simulink model "AFS_VDDrftComp"  (R2016b)
settings: configuration reference "CodeGenConfigSet" (kept outside this file)
values from neighbouring files (symbols this model uses):
  AFS_aOvrnAdjMax_C = Calibration.Parameter    [init_AFS_VDDrftComp.m]    (also in init_AFS_VDDrftComp_SIL.m = Simulink.Parameter)
  AFS_aOvrnAdjMin_C = Calibration.Parameter    [init_AFS_VDDrftComp.m]    (also in init_AFS_VDDrftComp_SIL.m = Simulink.Parameter)
  AFS_dmIdlAirMsLim_C = Calibration.Parameter    [init_AFS_VDDrftComp.m]    (also in init_AFS_VDDrftComp_SIL.m = Simulink.Parameter)
  AFS_dmLdAirMsLim_C = Calibration.Parameter    [init_AFS_VDDrftComp.m]    (also in init_AFS_VDDrftComp_SIL.m = Simulink.Parameter)
  AFS_dnEngLdAdjThresHi_C = Calibration.Parameter    [init_AFS_VDDrftComp.m]    (also in init_AFS_VDDrftComp_SIL.m = Simulink.Parameter)
  AFS_dpLdAdjThresHi_C = Calibration.Parameter    [init_AFS_VDDrftComp.m]    (also in init_AFS_VDDrftComp_SIL.m = Simulink.Parameter)
  AFS_dqLdAdjThresHi_C = Calibration.Parameter    [init_AFS_VDDrftComp.m]    (also in init_AFS_VDDrftComp_SIL.m = Simulink.Parameter)
  AFS_drWtPenDetThresHi_C = Calibration.Parameter    [init_AFS_VDDrftComp.m]    (also in init_AFS_VDDrftComp_SIL.m = Simulink.Parameter)
  AFS_facAdjPlausDiff_C = Calibration.Parameter    [init_AFS_VDDrftComp.m]    (also in init_AFS_VDDrftComp_SIL.m = Simulink.Parameter)
  AFS_facAirMsPT1_C = Calibration.Parameter    [init_AFS_VDDrftComp.m]    (also in init_AFS_VDDrftComp_SIL.m = Simulink.Parameter)
  AFS_facBstPresPT1_C = Calibration.Parameter    [init_AFS_VDDrftComp.m]    (also in init_AFS_VDDrftComp_SIL.m = Simulink.Parameter)
  AFS_facCorExtpIdl_CUR = Calibration.Parameter    [init_AFS_VDDrftComp.m]    (also in init_AFS_VDDrftComp_SIL.m = Simulink.Parameter)
  AFS_facCorExtpIdl_CURX = Calibration.Parameter    [init_AFS_VDDrftComp.m]    (also in init_AFS_VDDrftComp_SIL.m = Simulink.Parameter)
  AFS_facCorExtpLd_CUR = Calibration.Parameter    [init_AFS_VDDrftComp.m]    (also in init_AFS_VDDrftComp_SIL.m = Simulink.Parameter)
  AFS_facCorExtpLd_CURX = Calibration.Parameter    [init_AFS_VDDrftComp.m]    (also in init_AFS_VDDrftComp_SIL.m = Simulink.Parameter)
  AFS_facCorFacPT1_C = Calibration.Parameter    [init_AFS_VDDrftComp.m]    (also in init_AFS_VDDrftComp_SIL.m = Simulink.Parameter)
  AFS_facIdlAdjPlausMax_C = Calibration.Parameter    [init_AFS_VDDrftComp.m]    (also in init_AFS_VDDrftComp_SIL.m = Simulink.Parameter)
  AFS_facIdlAdjValMax_C = Calibration.Parameter    [init_AFS_VDDrftComp.m]    (also in init_AFS_VDDrftComp_SIL.m = Simulink.Parameter)
  AFS_facIdlAdjValMin_C = Calibration.Parameter    [init_AFS_VDDrftComp.m]    (also in init_AFS_VDDrftComp_SIL.m = Simulink.Parameter)
  AFS_facIdlAdjValStepLim_C = Calibration.Parameter    [init_AFS_VDDrftComp.m]    (also in init_AFS_VDDrftComp_SIL.m = Simulink.Parameter)
  AFS_facLdAdjPlausMin_C = Calibration.Parameter    [init_AFS_VDDrftComp.m]    (also in init_AFS_VDDrftComp_SIL.m = Simulink.Parameter)
  AFS_facLdAdjValMax_C = Calibration.Parameter    [init_AFS_VDDrftComp.m]    (also in init_AFS_VDDrftComp_SIL.m = Simulink.Parameter)
  AFS_facLdAdjValMin_C = Calibration.Parameter    [init_AFS_VDDrftComp.m]    (also in init_AFS_VDDrftComp_SIL.m = Simulink.Parameter)
  AFS_facLdAdjValStepLim_C = Calibration.Parameter    [init_AFS_VDDrftComp.m]    (also in init_AFS_VDDrftComp_SIL.m = Simulink.Parameter)
  AFS_facLoThresIdlAdjVal_C = Calibration.Parameter    [init_AFS_VDDrftComp.m]    (also in init_AFS_VDDrftComp_SIL.m = Simulink.Parameter)
  AFS_facLoThresLdAdjVal_C = Calibration.Parameter    [init_AFS_VDDrftComp.m]    (also in init_AFS_VDDrftComp_SIL.m = Simulink.Parameter)
  AFS_facnEngPT1_C = Calibration.Parameter    [init_AFS_VDDrftComp.m]    (also in init_AFS_VDDrftComp_SIL.m = Simulink.Parameter)
  AFS_facQntCurrPT1_C = Calibration.Parameter    [init_AFS_VDDrftComp.m]    (also in init_AFS_VDDrftComp_SIL.m = Simulink.Parameter)
  AFS_facWtPenDetPT1_C = Calibration.Parameter    [init_AFS_VDDrftComp.m]    (also in init_AFS_VDDrftComp_SIL.m = Simulink.Parameter)
  AFS_nAvrgIdlAdjThresHi_C = Calibration.Parameter    [init_AFS_VDDrftComp.m]    (also in init_AFS_VDDrftComp_SIL.m = Simulink.Parameter)
  AFS_nAvrgIdlAdjThresLo_C = Calibration.Parameter    [init_AFS_VDDrftComp.m]    (also in init_AFS_VDDrftComp_SIL.m = Simulink.Parameter)
  AFS_nOvrnAdjMax_C = Calibration.Parameter    [init_AFS_VDDrftComp.m]    (also in init_AFS_VDDrftComp_SIL.m = Simulink.Parameter)
  AFS_nOvrnAdjMin_C = Calibration.Parameter    [init_AFS_VDDrftComp.m]    (also in init_AFS_VDDrftComp_SIL.m = Simulink.Parameter)
  AFS_numAirDrftComp_C = Calibration.Parameter    [init_AFS_VDDrftComp.m]    (also in init_AFS_VDDrftComp_SIL.m = Simulink.Parameter)
  AFS_numEnvTemp_C = Calibration.Parameter    [init_AFS_VDDrftComp.m]    (also in init_AFS_VDDrftComp_SIL.m = Simulink.Parameter)
  AFS_numOvrnAdjGearMin_C = Calibration.Parameter    [init_AFS_VDDrftComp.m]    (also in init_AFS_VDDrftComp_SIL.m = Simulink.Parameter)
  AFS_pBstAtmDiffLim_C = Calibration.Parameter    [init_AFS_VDDrftComp.m]    (also in init_AFS_VDDrftComp_SIL.m = Simulink.Parameter)
  AFS_pBstLdAdjThresHi_C = Calibration.Parameter    [init_AFS_VDDrftComp.m]    (also in init_AFS_VDDrftComp_SIL.m = Simulink.Parameter)
  AFS_pBstLdAdjThresLo_C = Calibration.Parameter    [init_AFS_VDDrftComp.m]    (also in init_AFS_VDDrftComp_SIL.m = Simulink.Parameter)
  AFS_qCurrIdlAdjThresHi_C = Calibration.Parameter    [init_AFS_VDDrftComp.m]    (also in init_AFS_VDDrftComp_SIL.m = Simulink.Parameter)
  AFS_qCurrIdlAdjThresLo_C = Calibration.Parameter    [init_AFS_VDDrftComp.m]    (also in init_AFS_VDDrftComp_SIL.m = Simulink.Parameter)
  AFS_qWinLdAdjThresHi_CUR = Calibration.Parameter    [init_AFS_VDDrftComp.m]    (also in init_AFS_VDDrftComp_SIL.m = Simulink.Parameter)
  AFS_qWinLdAdjThresHi_CURX = Calibration.Parameter    [init_AFS_VDDrftComp.m]    (also in init_AFS_VDDrftComp_SIL.m = Simulink.Parameter)
  AFS_qWinLdAdjThresLo_CUR = Calibration.Parameter    [init_AFS_VDDrftComp.m]    (also in init_AFS_VDDrftComp_SIL.m = Simulink.Parameter)
  AFS_qWinLdAdjThresLo_CURX = Calibration.Parameter    [init_AFS_VDDrftComp.m]    (also in init_AFS_VDDrftComp_SIL.m = Simulink.Parameter)
  AFS_swtAdjPlausLim_C = Calibration.Parameter    [init_AFS_VDDrftComp.m]    (also in init_AFS_VDDrftComp_SIL.m = Simulink.Parameter)
  AFS_swtAirMsCorRls_C = Calibration.Parameter    [init_AFS_VDDrftComp.m]    (also in init_AFS_VDDrftComp_SIL.m = Simulink.Parameter)
  AFS_swtLdAdjSel_C = Calibration.Parameter    [init_AFS_VDDrftComp.m]    (also in init_AFS_VDDrftComp_SIL.m = Simulink.Parameter)
  AFS_tAirAdjRlsThresHi_C = Calibration.Parameter    [init_AFS_VDDrftComp.m]    (also in init_AFS_VDDrftComp_SIL.m = Simulink.Parameter)
  AFS_tAirAdjRlsThresLo_C = Calibration.Parameter    [init_AFS_VDDrftComp.m]    (also in init_AFS_VDDrftComp_SIL.m = Simulink.Parameter)
  AFS_tEnvAdjRlsThresHi_C = Calibration.Parameter    [init_AFS_VDDrftComp.m]    (also in init_AFS_VDDrftComp_SIL.m = Simulink.Parameter)
  AFS_tEnvAdjRlsThresLo_C = Calibration.Parameter    [init_AFS_VDDrftComp.m]    (also in init_AFS_VDDrftComp_SIL.m = Simulink.Parameter)
  AFS_tiAdjRlsDel_C = Calibration.Parameter    [init_AFS_VDDrftComp.m]    (also in init_AFS_VDDrftComp_SIL.m = Simulink.Parameter)
  AFS_tiIdlAdjRlsDeb = Calibration.Parameter    [init_AFS_VDDrftComp.m]    (also in init_AFS_VDDrftComp_SIL.m = Simulink.Parameter)
  AFS_tiLdAdjRlsDeb = Calibration.Parameter    [init_AFS_VDDrftComp.m]    (also in init_AFS_VDDrftComp_SIL.m = Simulink.Parameter)
  AFS_tiStrtDelAdjRls_C = Calibration.Parameter    [init_AFS_VDDrftComp.m]    (also in init_AFS_VDDrftComp_SIL.m = Simulink.Parameter)
  AFS_tiWtPenDeb = Calibration.Parameter    [init_AFS_VDDrftComp.m]    (also in init_AFS_VDDrftComp_SIL.m = Simulink.Parameter)
  AFS_vOvrnAdjMin_C = Calibration.Parameter    [init_AFS_VDDrftComp.m]    (also in init_AFS_VDDrftComp_SIL.m = Simulink.Parameter)
  AFS_vVehLdAdjThresHi_C = Calibration.Parameter    [init_AFS_VDDrftComp.m]    (also in init_AFS_VDDrftComp_SIL.m = Simulink.Parameter)
  AFS_vVehLdAdjThresLo_C = Calibration.Parameter    [init_AFS_VDDrftComp.m]    (also in init_AFS_VDDrftComp_SIL.m = Simulink.Parameter)
  AIRCTL_DRFTCOMP = fi(5,State_uint8)    [init_AFS_VDDrftComp.m]    (also in init_AFS_VDDrftComp_SIL.m)
undefined symbols (not defined in the file or in its folder): AFS_VDDrftComp_DT, Switch_conv
libraries: simulink x82, CXLib x13
(part 1 of 2)
settings Model: Creator=Colin  LastModifiedBy=guanxiaoxing
settings ConfigSetRef: SourceLocation=Base Workspace

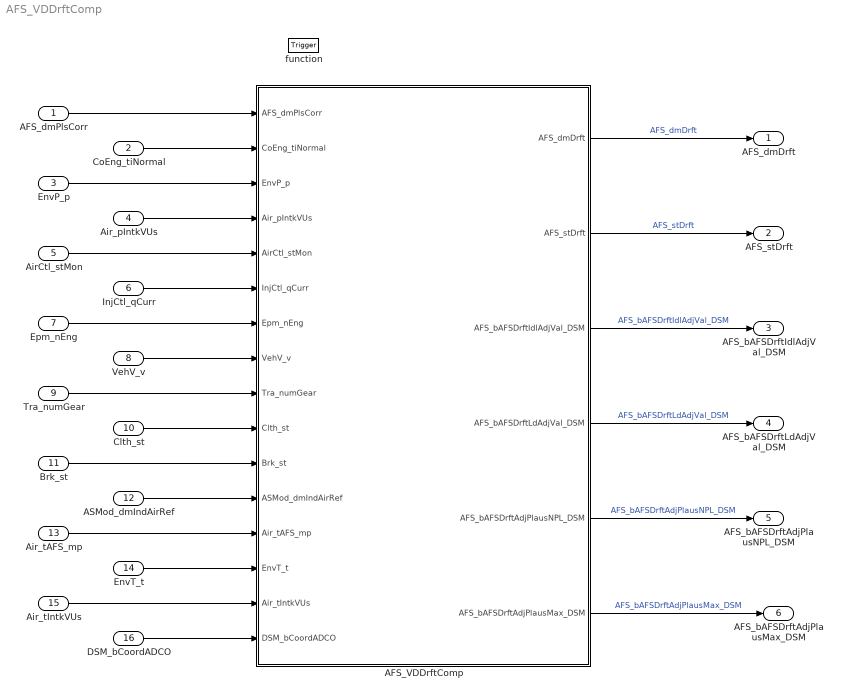
== system AFS_VDDrftComp ==
  AFS_dmPlsCorr : Inport  Tag=kg/h  Description=Pulsation corrected air mass.  OutMin=-8192  OutMax=8191  OutDataTypeStr=AirMassPerTime
  CoEng_tiNormal : Inport  Tag=ms  Description="Time since state\"CONENG_RUNNING\"was reached"  Port=2  OutMin=0  OutMax=42949672950  OutDataTypeStr=EngTime_ms
  EnvP_p : Inport  Tag=kPa  Description=Barometric pressure  Port=3  OutMin=0  OutMax=3276  OutDataTypeStr=AirPressure_kPa
  Air_pIntkVUs : Inport  Tag=kPa  Description=Intake valve upstream pressure  Port=4  OutMin=0  OutMax=1200  OutDataTypeStr=AirPressure_kPa
  AirCtl_stMon : Inport  Description=status: shutdown case of the governor  Port=5  OutMin=0  OutMax=255  OutDataTypeStr=State_uint8
  InjCtl_qCurr : Inport  Tag=mg/hub  Description=Torque generating engine fuel injection quantity  Port=6  OutMin=-319  OutMax=319  OutDataTypeStr=FuelMass_mg_hub
  Epm_nEng : Inport  Tag=rpm  Description=Engine speed  Port=7  OutMin=0  OutMax=6000  OutDataTypeStr=EngSpeed_rpm
  VehV_v : Inport  Tag=km/h  Description=Vehicle speed  Port=8  OutMin=0  OutMax=250  OutDataTypeStr=VehSpeed_km_h
  Tra_numGear : Inport  Description=Current gear information  Port=9  OutMin=-128  OutMax=127  OutDataTypeStr=Tra_num
  Clth_st : Inport  Description=Clutch information  Port=10  OutMin=0  OutMax=255  OutDataTypeStr=State_uint8
  Brk_st : Inport  Description=Brake switch state  Port=11  OutMin=0  OutMax=255  OutDataTypeStr=State_uint8
  ASMod_dmIndAirRef : Inport  Tag=kg/h  Description=Reference of gas mass flow into the engine while exhaust-gas recirculation is closed  Port=12  OutMin=-8192  OutMax=8191  OutDataTypeStr=AirMassPerTime
  Air_tAFS_mp : Inport  Tag=deg  Description=Induction air temperature at the HFM  Port=13  OutMin=-200  OutMax=200  OutDataTypeStr=Temp_deg
  EnvT_t : Inport  Tag=deg  Description=Environmental temperature  Port=14  OutMin=-200  OutMax=200  OutDataTypeStr=Temp_deg
  Air_tIntkVUs : Inport  Tag=deg  Description=Intake air temperature upstream of the inlet valve  Port=15  OutMin=-200  OutMax=200  OutDataTypeStr=Temp_deg
  DSM_bCoordADCO : Inport  Description="Release conditions for Overrun Coordinator\""  Port=16  OutMin=0  OutMax=1  OutDataTypeStr=boolean
  function : TriggerPort  TriggerType=function-call  VariantControl=Variant
  AFS_VDDrftComp : Subsystem
  AFS_dmDrft : Outport  Tag=kg/h  Description=Compensated Air mass value for the drift  OutMin=-8192  OutMax=8191  OutDataTypeStr=AirMassPerTime
  AFS_stDrft : Outport  Description=Status of drift compensation  Port=2  OutMin=0  OutMax=255  OutDataTypeStr=State_uint8
  AFS_bAFSDrftIdlAdjVal_DSM : Outport  Description=fault flag for low idle correction factor exceeding the maximum drift limit  Port=3  OutMin=0  OutMax=1  OutDataTypeStr=boolean
  AFS_bAFSDrftLdAdjVal_DSM : Outport  Description=fault flag for load correction factor exceeding the maximum drift limit  Port=4  OutMin=0  OutMax=1  OutDataTypeStr=boolean
  AFS_bAFSDrftAdjPlausNPL_DSM : Outport  Description=fault flag for Maximum Difference Plausibility of Drift Adjustment  Port=5  OutMin=0  OutMax=1  OutDataTypeStr=boolean
  AFS_bAFSDrftAdjPlausMax_DSM : Outport  Description=fault flag for Plausibility of Drift Adjustment  Port=6  OutMin=0  OutMax=1  OutDataTypeStr=boolean
  wires:
  AFS_VDDrftComp/1(AFS_dmDrft) -> AFS_dmDrft/1  "AFS_dmDrft"
  AFS_VDDrftComp/2(AFS_stDrft) -> AFS_stDrft/1  "AFS_stDrft"
  AFS_dmPlsCorr/1 -> AFS_VDDrftComp/1(AFS_dmPlsCorr)
  CoEng_tiNormal/1 -> AFS_VDDrftComp/2(CoEng_tiNormal)
  EnvP_p/1 -> AFS_VDDrftComp/3(EnvP_p)
  Air_pIntkVUs/1 -> AFS_VDDrftComp/4(Air_pIntkVUs)
  AirCtl_stMon/1 -> AFS_VDDrftComp/5(AirCtl_stMon)
  VehV_v/1 -> AFS_VDDrftComp/8(VehV_v)
  Tra_numGear/1 -> AFS_VDDrftComp/9(Tra_numGear)
  Clth_st/1 -> AFS_VDDrftComp/10(Clth_st)
  Brk_st/1 -> AFS_VDDrftComp/11(Brk_st)
  InjCtl_qCurr/1 -> AFS_VDDrftComp/6(InjCtl_qCurr)
  ASMod_dmIndAirRef/1 -> AFS_VDDrftComp/12(ASMod_dmIndAirRef)
  Epm_nEng/1 -> AFS_VDDrftComp/7(Epm_nEng)
  Air_tAFS_mp/1 -> AFS_VDDrftComp/13(Air_tAFS_mp)
  EnvT_t/1 -> AFS_VDDrftComp/14(EnvT_t)
  Air_tIntkVUs/1 -> AFS_VDDrftComp/15(Air_tIntkVUs)
  DSM_bCoordADCO/1 -> AFS_VDDrftComp/16(DSM_bCoordADCO)
  AFS_VDDrftComp/3(AFS_bAFSDrftIdlAdjVal_DSM) -> AFS_bAFSDrftIdlAdjVal_DSM/1  "AFS_bAFSDrftIdlAdjVal_DSM"
  AFS_VDDrftComp/4(AFS_bAFSDrftLdAdjVal_DSM) -> AFS_bAFSDrftLdAdjVal_DSM/1  "AFS_bAFSDrftLdAdjVal_DSM"
  AFS_VDDrftComp/5(AFS_bAFSDrftAdjPlausNPL_DSM) -> AFS_bAFSDrftAdjPlausNPL_DSM/1  "AFS_bAFSDrftAdjPlausNPL_DSM"
  AFS_VDDrftComp/6(AFS_bAFSDrftAdjPlausMax_DSM) -> AFS_bAFSDrftAdjPlausMax_DSM/1  "AFS_bAFSDrftAdjPlausMax_DSM"

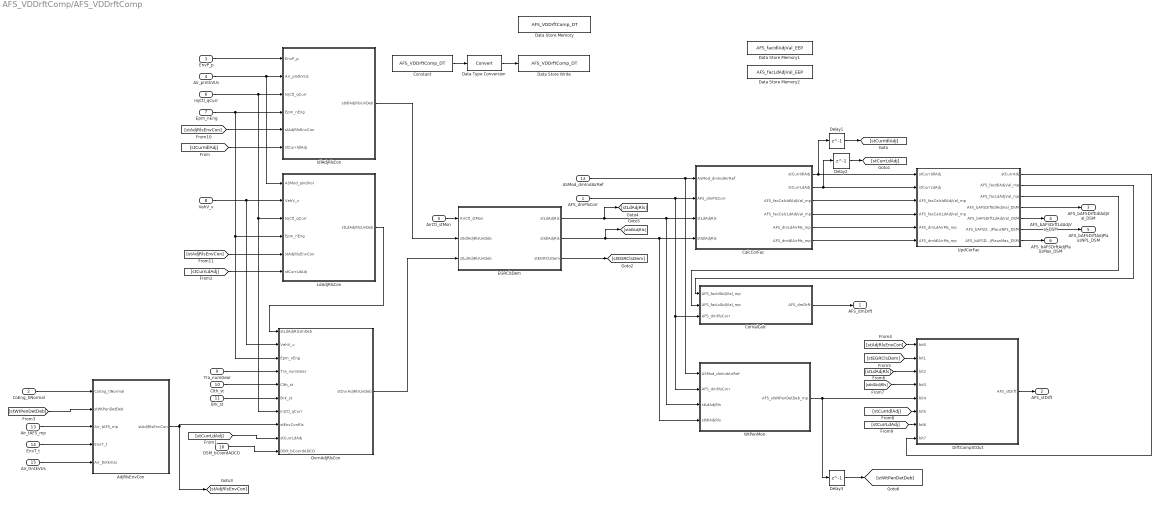
== system AFS_VDDrftComp/AFS_VDDrftComp ==
  AFS_dmPlsCorr : Inport
  CoEng_tiNormal : Inport  Port=2
  EnvP_p : Inport  Port=3
  Air_pIntkVUs : Inport  Port=4
  AirCtl_stMon : Inport  Port=5
  InjCtl_qCurr : Inport  Port=6
  Epm_nEng : Inport  Port=7
  VehV_v : Inport  Port=8
  Tra_numGear : Inport  Port=9
  Clth_st : Inport  Port=10
  Brk_st : Inport  Port=11
  ASMod_dmIndAirRef : Inport  Port=12
  Air_tAFS_mp : Inport  Port=13
  EnvT_t : Inport  Port=14
  Air_tIntkVUs : Inport  Port=15
  DSM_bCoordADCO : Inport  Port=16
  " AdjRlsEnvCon" : Subsystem
  " IdlAdjRlsCon" : Subsystem
  " LdAdjRlsCon" : Subsystem
  CalcCorFac : Subsystem
  Constant : Constant  Value=AFS_VDDrftComp_DT
  CorValCalc : Subsystem
  Data Store Memory : DataStoreMemory  DataStoreName=AFS_VDDrftComp_DT  ReadBeforeWriteMsg=warning  WriteAfterWriteMsg=warning  WriteAfterReadMsg=warning  ShowAdditionalParam=off
  Data Store Memory1 : DataStoreMemory  DataStoreName=AFS_facIdlAdjVal_EEP  ReadBeforeWriteMsg=warning  WriteAfterWriteMsg=warning  WriteAfterReadMsg=warning  ShowAdditionalParam=off
  Data Store Memory2 : DataStoreMemory  DataStoreName=AFS_facLdAdjVal_EEP  ReadBeforeWriteMsg=warning  WriteAfterWriteMsg=warning  WriteAfterReadMsg=warning  ShowAdditionalParam=off
  Data Store Write : DataStoreWrite  DataStoreName=AFS_VDDrftComp_DT
  Data Type Conversion : DataTypeConversion
  Delay1 : Delay  DelayLength=1  InitialCondition=0
  Delay2 : Delay  DelayLength=1  InitialCondition=0
  Delay3 : Delay  DelayLength=1  InitialCondition=0
  DrftCompStOut : Subsystem
  EGRClsDem : Subsystem
  OvrnAdjRlsCon : Subsystem
  UpdCorFac : Subsystem
  WtPenMon : Subsystem
  AFS_dmDrft : Outport
  AFS_stDrft : Outport  Port=2
  AFS_bAFSDrftIdlAdjVal_DSM : Outport  Port=3
  AFS_bAFSDrftLdAdjVal_DSM : Outport  Port=4
  AFS_bAFSDrftAdjPlausNPL_DSM : Outport  Port=5
  AFS_bAFSDrftAdjPlausMax_DSM : Outport  Port=6
  wires:
  OvrnAdjRlsCon/1(stOvrAdjRlsUnDeb) -> EGRClsDem/3(stLdAdjRlsUnDeb)
  " LdAdjRlsCon"/1(stLdAdjRlsUnDeb) -> OvrnAdjRlsCon/1(stLdAdjRlsUnDeb)
  " IdlAdjRlsCon"/1(stIdlAdjRlsUnDeb) -> EGRClsDem/2(stIdlAdjRlsUnDeb)
  Tra_numGear/1 -> OvrnAdjRlsCon/4(Tra_numGear)
  Clth_st/1 -> OvrnAdjRlsCon/5(Clth_st)
  VehV_v/1 -> OvrnAdjRlsCon/2(VehV_v), " LdAdjRlsCon"/2(VehV_v)
  Brk_st/1 -> OvrnAdjRlsCon/6(Brk_st)
  Epm_nEng/1 -> OvrnAdjRlsCon/3(Epm_nEng), " LdAdjRlsCon"/4(Epm_nEng), " IdlAdjRlsCon"/4(Epm_nEng)
  EGRClsDem/1(stLdAdjRls) -> [stLdAdjRls], CalcCorFac/3(stLdAdjRls), WtPenMon/3(stLdAdjRls)
  InjCtl_qCurr/1 -> OvrnAdjRlsCon/7(InjCtl_qCurr), " LdAdjRlsCon"/3(InjCtl_qCurr), " IdlAdjRlsCon"/3(InjCtl_qCurr)
  EGRClsDem/2(stIdlAdjRls) -> [stIdlAdjRls], CalcCorFac/4(stIdlAdjRls), WtPenMon/4(stIdlAdjRls)
  [stCurrLdAdj] -> " LdAdjRlsCon"/6(stCurrLdAdj)
  WtPenMon/1(AFS_stWtPenDetDeb_mp) -> Delay3/1, DrftCompStOut/5(bit4)
  [stIdlAdjRls] -> DrftCompStOut/4(bit3)
  CoEng_tiNormal/1 -> " AdjRlsEnvCon"/1(CoEng_tiNormal)
  [stWtPenDetDeb] -> " AdjRlsEnvCon"/2(stWtPenDetDeb)
  " AdjRlsEnvCon"/1(stAdjRlsEnvCon) -> OvrnAdjRlsCon/8(stEnvConRls), [stAdjRlsEnvCon]
  EnvP_p/1 -> " IdlAdjRlsCon"/1(EnvP_p)
  Air_pIntkVUs/1 -> " LdAdjRlsCon"/1(ASMod_pIndVol), " IdlAdjRlsCon"/2(Air_pIntkVUs)
  [stLdAdjRls] -> DrftCompStOut/3(bit2)
  [stAdjRlsEnvCon] -> DrftCompStOut/1(bit0)
  [stEGRClsDem] -> DrftCompStOut/2(bit1)
  DrftCompStOut/1(AFS_stDrft) -> AFS_stDrft/1
  UpdCorFac/1(stCurrAdj) -> DrftCompStOut/8(bit7)
  AFS_dmPlsCorr/1 -> CalcCorFac/2(AFS_dmPlsCorr), WtPenMon/2(AFS_dmPlsCorr), CorValCalc/3(AFS_dmPlsCorr)
  CalcCorFac/4(AFS_facCalcLdAdjVal_mp) -> UpdCorFac/4(AFS_facCalcLdAdjVal_mp)
  ASMod_dmIndAirRef/1 -> CalcCorFac/1(ASMod_dmIndAirRef), WtPenMon/1(ASMod_dmIndAirRef)
  CalcCorFac/5(AFS_dmLdAirMs_mp) -> UpdCorFac/5(AFS_dmLdAirMs_mp)
  CalcCorFac/6(AFS_dmIdlAirMs_mp) -> UpdCorFac/6(AFS_dmIdlAirMs_mp)
  CalcCorFac/3(AFS_facCalcIdlAdjVal_mp) -> UpdCorFac/3(AFS_facCalcIdlAdjVal_mp)
  CorValCalc/1(AFS_dmDrft) -> AFS_dmDrft/1
  [stCurrIdlAdj] -> " IdlAdjRlsCon"/6(stCurrIdlAdj)
  [stCurrLdAdj] -> OvrnAdjRlsCon/9(stCurrLdAdj)
  [stCurrIdlAdj] -> DrftCompStOut/6(bit5)
  [stCurrLdAdj] -> DrftCompStOut/7(bit6)
  AirCtl_stMon/1 -> EGRClsDem/1(AirCtl_stMon)
  CalcCorFac/1(stCurrIdlAdj) -> Delay1/1, UpdCorFac/1(stCurrIdlAdj)
  CalcCorFac/2(stCurrLdAdj) -> Delay2/1, UpdCorFac/2(stCurrLdAdj)
  EGRClsDem/3(stEGRClsDem) -> [stEGRClsDem]
  [stAdjRlsEnvCon] -> " IdlAdjRlsCon"/5(stAdjRlsEnvCon)
  [stAdjRlsEnvCon] -> " LdAdjRlsCon"/5(stAdjRlsEnvCon)
  UpdCorFac/3(AFS_facLdAdjVal_mp) -> CorValCalc/2(AFS_facLdAdjVal_mp)
  UpdCorFac/2(AFS_facIdlAdjVal_mp) -> CorValCalc/1(AFS_facIdlAdjVal_mp)
  Air_tAFS_mp/1 -> " AdjRlsEnvCon"/3(Air_tAFS_mp)
  EnvT_t/1 -> " AdjRlsEnvCon"/4(EnvT_t)
  Air_tIntkVUs/1 -> " AdjRlsEnvCon"/5(Air_tIntkVUs)
  Constant/1 -> Data Type Conversion/1
  DSM_bCoordADCO/1 -> OvrnAdjRlsCon/10(DSM_bCoordADCO)
  Delay3/1 -> [stWtPenDetDeb]
  UpdCorFac/4(AFS_bAFSDrftIdlAdjVal_DSM) -> AFS_bAFSDrftIdlAdjVal_DSM/1
  UpdCorFac/5(AFS_bAFSDrftLdAdjVal_DSM) -> AFS_bAFSDrftLdAdjVal_DSM/1
  UpdCorFac/6(AFS_bAFSDrftAdjPlausNPL_DSM) -> AFS_bAFSDrftAdjPlausNPL_DSM/1
  UpdCorFac/7(AFS_bAFSDrftAdjPlausMax_DSM) -> AFS_bAFSDrftAdjPlausMax_DSM/1
  Delay1/1 -> [stCurrIdlAdj]
  Delay2/1 -> [stCurrLdAdj]
  Data Type Conversion/1 -> Data Store Write/1

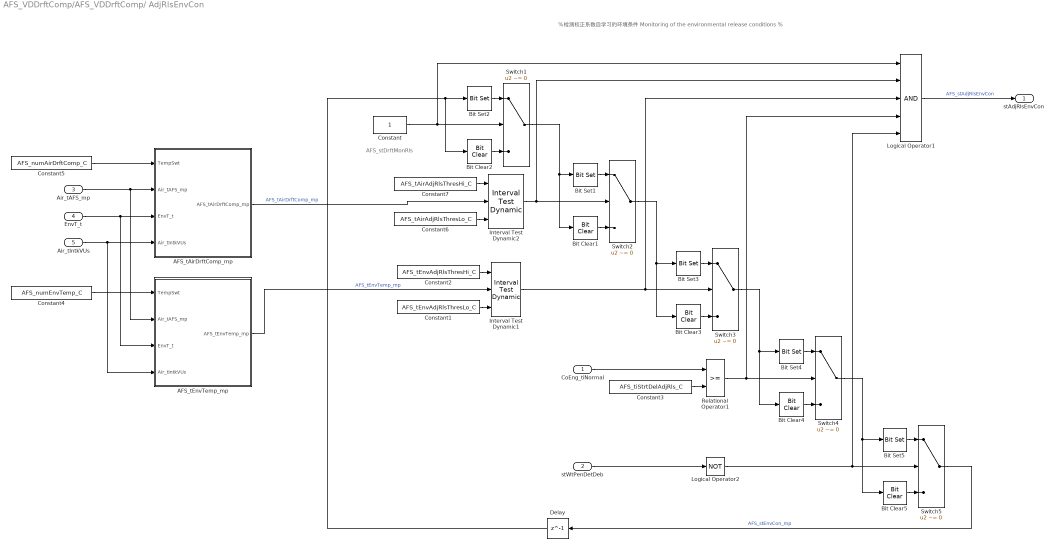
== system AFS_VDDrftComp/AFS_VDDrftComp/ AdjRlsEnvCon ==
  note: AFS_stDrftMonRls
  note: %检测校正系数自学习的环境条件
      | Monitoring of the environmental release conditions %
  CoEng_tiNormal : Inport
  stWtPenDetDeb : Inport  Port=2
  Air_tAFS_mp : Inport  Tag=deg  Description=Induction air temperature at the HFM  Port=3  OutMin=-200  OutMax=200  OutDataTypeStr=Temp_deg
  EnvT_t : Inport  Tag=deg  Description=Environmental temperature  Port=4  OutMin=-200  OutMax=200  OutDataTypeStr=Temp_deg
  Air_tIntkVUs : Inport  Tag=deg  Description=Intake air temperature upstream of the inlet valve  Port=5  OutMin=-200  OutMax=200  OutDataTypeStr=Temp_deg
  AFS_tAirDrftComp_mp : Subsystem
  AFS_tEnvTemp_mp : Subsystem
  Bit Clear1 : simulink/Logic and Bit Operations/Bit Clear  iBit=1
  Bit Clear2 : simulink/Logic and Bit Operations/Bit Clear  iBit=0
  Bit Clear3 : simulink/Logic and Bit Operations/Bit Clear  iBit=2
  Bit Clear4 : simulink/Logic and Bit Operations/Bit Clear  iBit=3
  Bit Clear5 : simulink/Logic and Bit Operations/Bit Clear  iBit=4
  Bit Set1 : simulink/Logic and Bit Operations/Bit Set  iBit=1
  Bit Set2 : simulink/Logic and Bit Operations/Bit Set  iBit=0
  Bit Set3 : simulink/Logic and Bit Operations/Bit Set  iBit=2
  Bit Set4 : simulink/Logic and Bit Operations/Bit Set  iBit=3
  Bit Set5 : simulink/Logic and Bit Operations/Bit Set  iBit=4
  Constant : Constant  OutDataTypeStr=boolean
  Constant1 : Constant  Value=AFS_tEnvAdjRlsThresLo_C
  Constant2 : Constant  Value=AFS_tEnvAdjRlsThresHi_C
  Constant3 : Constant  Value=AFS_tiStrtDelAdjRls_C
  Constant4 : Constant  Value=AFS_numEnvTemp_C
  Constant5 : Constant  Value=AFS_numAirDrftComp_C
  Constant6 : Constant  Value=AFS_tAirAdjRlsThresLo_C
  Constant7 : Constant  Value=AFS_tAirAdjRlsThresHi_C
  Delay : Delay  DelayLength=1  InitialCondition=0
  Interval Test Dynamic1 : simulink/Logic and Bit Operations/Interval Test Dynamic  IntervalClosedRight=off  IntervalClosedLeft=off  OutDataTypeStr=boolean
  Interval Test Dynamic2 : simulink/Logic and Bit Operations/Interval Test Dynamic  IntervalClosedRight=off  IntervalClosedLeft=off  OutDataTypeStr=boolean
  Logical Operator1 : Logic  Inputs=5  AllPortsSameDT=off  OutDataTypeStr=boolean
  Logical Operator2 : Logic  Operator=NOT  Inputs=5  AllPortsSameDT=off  OutDataTypeStr=boolean
  Relational Operator1 : RelationalOperator  OutDataTypeStr=boolean  RndMeth=Nearest  InputSameDT=on
  Switch{1..5} (5 alike) : Switch  Criteria=u2 ~= 0  OutDataTypeStr=Inherit: Inherit via back propagation  SaturateOnIntegerOverflow=on  InputSameDT=on
  stAdjRlsEnvCon : Outport
  wires:
  Constant4/1 -> AFS_tEnvTemp_mp/1(TempSwt)
  AFS_tEnvTemp_mp/1(AFS_tEnvTemp_mp) -> Interval Test Dynamic1/2  "AFS_tEnvTemp_mp"
  AFS_tAirDrftComp_mp/1(AFS_tAirDrftComp_mp) -> Interval Test Dynamic2/2  "AFS_tAirDrftComp_mp"
  Bit Clear4/1 -> Switch4/3
  Relational Operator1/1 -> Switch4/2, Logical Operator1/4
  Bit Set4/1 -> Switch4/1
  Switch3/1 -> Bit Set4/1, Bit Clear4/1
  Logical Operator1/1 -> stAdjRlsEnvCon/1  "AFS_stAdjRlsEnvCon"
  Switch5/1 -> Delay/1  "AFS_stEnvCon_mp"
  Constant3/1 -> Relational Operator1/2
  Constant2/1 -> Interval Test Dynamic1/1
  Interval Test Dynamic1/1 -> Switch3/2, Logical Operator1/3
  Constant1/1 -> Interval Test Dynamic1/3
  Switch2/1 -> Bit Clear3/1, Bit Set3/1
  CoEng_tiNormal/1 -> Relational Operator1/1
  Bit Set3/1 -> Switch3/1
  Bit Clear3/1 -> Switch3/3
  Delay/1 -> Bit Set2/1, Bit Clear2/1
  Bit Set2/1 -> Switch1/1
  Bit Clear2/1 -> Switch1/3
  Switch1/1 -> Bit Set1/1, Bit Clear1/1
  stWtPenDetDeb/1 -> Logical Operator2/1
  Bit Set1/1 -> Switch2/1
  Bit Set5/1 -> Switch5/1
  Logical Operator2/1 -> Switch5/2, Logical Operator1/5
  Bit Clear5/1 -> Switch5/3
  Switch4/1 -> Bit Clear5/1, Bit Set5/1
  Interval Test Dynamic2/1 -> Switch2/2, Logical Operator1/2
  Constant7/1 -> Interval Test Dynamic2/1
  Constant/1 -> Switch1/2, Logical Operator1/1
  Bit Clear1/1 -> Switch2/3
  Constant6/1 -> Interval Test Dynamic2/3
  Constant5/1 -> AFS_tAirDrftComp_mp/1(TempSwt)
  Air_tAFS_mp/1 -> AFS_tEnvTemp_mp/2(Air_tAFS_mp), AFS_tAirDrftComp_mp/2(Air_tAFS_mp)
  EnvT_t/1 -> AFS_tEnvTemp_mp/3(EnvT_t), AFS_tAirDrftComp_mp/3(EnvT_t)
  Air_tIntkVUs/1 -> AFS_tEnvTemp_mp/4(Air_tIntkVUs), AFS_tAirDrftComp_mp/4(Air_tIntkVUs)

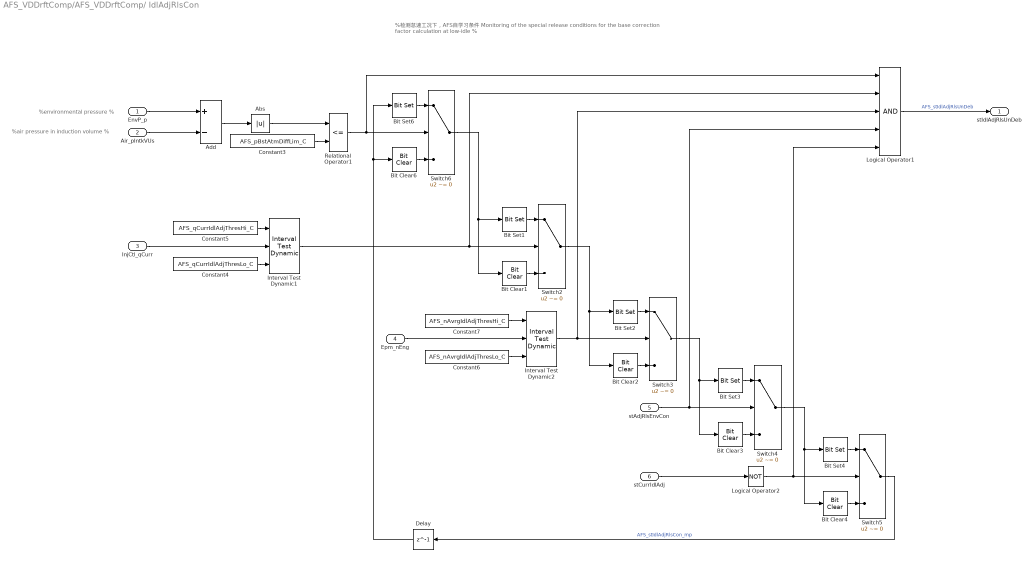
== system AFS_VDDrftComp/AFS_VDDrftComp/ IdlAdjRlsCon ==
  note: %检测怠速工况下，AFS自学习条件
      | Monitoring of the special release conditions for the base correction factor calculation at low-idle %
  note: %environmental pressure %
  note: %air pressure in induction volume %
  EnvP_p : Inport
  Air_pIntkVUs : Inport  Port=2
  InjCtl_qCurr : Inport  Port=3
  Epm_nEng : Inport  Port=4
  stAdjRlsEnvCon : Inport  Port=5
  stCurrIdlAdj : Inport  Port=6
  Abs : Abs  SaturateOnIntegerOverflow=on
  Add : Sum  Inputs=+-  OutDataTypeStr=Inherit: Inherit via back propagation  SaturateOnIntegerOverflow=on  InputSameDT=on
  Bit Clear1 : simulink/Logic and Bit Operations/Bit Clear  iBit=1
  Bit Clear2 : simulink/Logic and Bit Operations/Bit Clear  iBit=2
  Bit Clear3 : simulink/Logic and Bit Operations/Bit Clear  iBit=3
  Bit Clear4 : simulink/Logic and Bit Operations/Bit Clear  iBit=4
  Bit Clear6 : simulink/Logic and Bit Operations/Bit Clear  iBit=0
  Bit Set1 : simulink/Logic and Bit Operations/Bit Set  iBit=1
  Bit Set2 : simulink/Logic and Bit Operations/Bit Set  iBit=2
  Bit Set3 : simulink/Logic and Bit Operations/Bit Set  iBit=3
  Bit Set4 : simulink/Logic and Bit Operations/Bit Set  iBit=4
  Bit Set6 : simulink/Logic and Bit Operations/Bit Set  iBit=0
  Constant3 : Constant  Value=AFS_pBstAtmDiffLim_C
  Constant4 : Constant  Value=AFS_qCurrIdlAdjThresLo_C
  Constant5 : Constant  Value=AFS_qCurrIdlAdjThresHi_C
  Constant6 : Constant  Value=AFS_nAvrgIdlAdjThresLo_C
  Constant7 : Constant  Value=AFS_nAvrgIdlAdjThresHi_C
  Delay : Delay  DelayLength=1  InitialCondition=0
  Interval Test Dynamic1 : simulink/Logic and Bit Operations/Interval Test Dynamic  IntervalClosedRight=off  IntervalClosedLeft=off  OutDataTypeStr=boolean
  Interval Test Dynamic2 : simulink/Logic and Bit Operations/Interval Test Dynamic  IntervalClosedRight=off  IntervalClosedLeft=off  OutDataTypeStr=boolean
  Logical Operator1 : Logic  Inputs=5  AllPortsSameDT=off  OutDataTypeStr=boolean
  Logical Operator2 : Logic  Operator=NOT  Inputs=5  AllPortsSameDT=off  OutDataTypeStr=boolean
  Relational Operator1 : RelationalOperator  Operator=<=  OutDataTypeStr=boolean  RndMeth=Nearest  InputSameDT=on
  Switch{2..6} (5 alike) : Switch  Criteria=u2 ~= 0  OutDataTypeStr=Inherit: Inherit via back propagation  SaturateOnIntegerOverflow=on  InputSameDT=on
  stIdlAdjRlsUnDeb : Outport
  wires:
  Logical Operator1/1 -> stIdlAdjRlsUnDeb/1  "AFS_stIdlAdjRlsUnDeb"
  Switch5/1 -> Delay/1  "AFS_stIdlAdjRlsCon_mp"
  Logical Operator2/1 -> Switch5/2, Logical Operator1/5
  Bit Set4/1 -> Switch5/1
  Bit Clear4/1 -> Switch5/3
  Switch4/1 -> Bit Clear4/1, Bit Set4/1
  stCurrIdlAdj/1 -> Logical Operator2/1
  stAdjRlsEnvCon/1 -> Switch4/2, Logical Operator1/4
  Bit Set3/1 -> Switch4/1
  Bit Clear3/1 -> Switch4/3
  Switch3/1 -> Bit Set3/1, Bit Clear3/1
  Interval Test Dynamic2/1 -> Switch3/2, Logical Operator1/3
  Bit Set2/1 -> Switch3/1
  Bit Clear2/1 -> Switch3/3
  Switch2/1 -> Bit Set2/1, Bit Clear2/1
  Epm_nEng/1 -> Interval Test Dynamic2/2
  Constant6/1 -> Interval Test Dynamic2/3
  Constant7/1 -> Interval Test Dynamic2/1
  Interval Test Dynamic1/1 -> Switch2/2, Logical Operator1/2
  Bit Set1/1 -> Switch2/1
  Bit Clear1/1 -> Switch2/3
  Switch6/1 -> Bit Clear1/1, Bit Set1/1
  Relational Operator1/1 -> Switch6/2, Logical Operator1/1
  Bit Set6/1 -> Switch6/1
  Bit Clear6/1 -> Switch6/3
  Delay/1 -> Bit Clear6/1, Bit Set6/1
  Constant4/1 -> Interval Test Dynamic1/3
  Constant5/1 -> Interval Test Dynamic1/1
  InjCtl_qCurr/1 -> Interval Test Dynamic1/2
  Abs/1 -> Relational Operator1/1
  Constant3/1 -> Relational Operator1/2
  EnvP_p/1 -> Add/1
  Add/1 -> Abs/1
  Air_pIntkVUs/1 -> Add/2

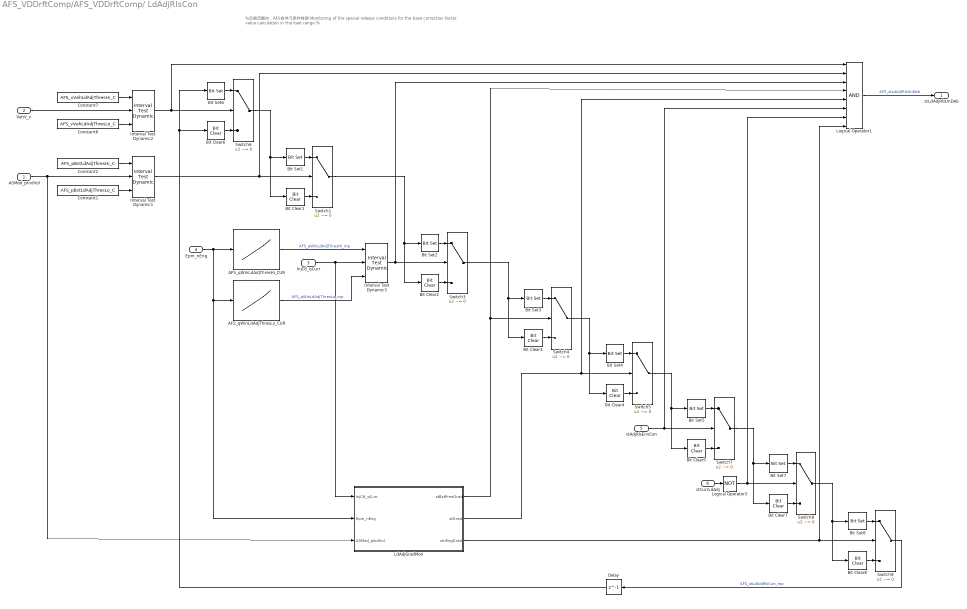
== system AFS_VDDrftComp/AFS_VDDrftComp/ LdAdjRlsCon ==
  note: %负载范围内，AFS自学习条件检测
      | Monitoring of the special release conditions for the base correction factor value calculation in the
      | load range %
  ASMod_pIndVol : Inport
  VehV_v : Inport  Port=2
  InjCtl_qCurr : Inport  Port=3
  Epm_nEng : Inport  Port=4
  stAdjRlsEnvCon : Inport  Port=5
  stCurrLdAdj : Inport  Port=6
  " LdAdjGradMon" : Subsystem
  AFS_qWinLdAdjThresHi_CUR : Lookup_n-D  NumberOfTableDimensions=1  BreakpointsForDimension1=AFS_qWinLdAdjThresHi_CURX  IndexSearchMethod=Linear search  BeginIndexSearchUsingPreviousIndexResult=on  UseOneInputPortForAllInputData=on  Table=AFS_qWinLdAdjThresHi_CUR  ExtrapMethod=Clip  UseLastTableValue=on  InternalRulePriority=Speed  OutDataTypeStr=Inherit: Inherit via back propagation  SaturateOnIntegerOverflow=on
  AFS_qWinLdAdjThresLo_CUR : Lookup_n-D  NumberOfTableDimensions=1  BreakpointsForDimension1=AFS_qWinLdAdjThresLo_CURX  IndexSearchMethod=Linear search  BeginIndexSearchUsingPreviousIndexResult=on  UseOneInputPortForAllInputData=on  Table=AFS_qWinLdAdjThresLo_CUR  ExtrapMethod=Clip  UseLastTableValue=on  InternalRulePriority=Speed  OutDataTypeStr=Inherit: Inherit via back propagation  SaturateOnIntegerOverflow=on
  Bit Clear1 : simulink/Logic and Bit Operations/Bit Clear  iBit=1
  Bit Clear2 : simulink/Logic and Bit Operations/Bit Clear  iBit=2
  Bit Clear3 : simulink/Logic and Bit Operations/Bit Clear  iBit=3
  Bit Clear4 : simulink/Logic and Bit Operations/Bit Clear  iBit=4
  Bit Clear5 : simulink/Logic and Bit Operations/Bit Clear  iBit=5
  Bit Clear6 : simulink/Logic and Bit Operations/Bit Clear  iBit=0
  Bit Clear7 : simulink/Logic and Bit Operations/Bit Clear  iBit=6
  Bit Clear8 : simulink/Logic and Bit Operations/Bit Clear  iBit=7
  Bit Set1 : simulink/Logic and Bit Operations/Bit Set  iBit=1
  Bit Set2 : simulink/Logic and Bit Operations/Bit Set  iBit=2
  Bit Set3 : simulink/Logic and Bit Operations/Bit Set  iBit=3
  Bit Set4 : simulink/Logic and Bit Operations/Bit Set  iBit=4
  Bit Set5 : simulink/Logic and Bit Operations/Bit Set  iBit=5
  Bit Set6 : simulink/Logic and Bit Operations/Bit Set  iBit=0
  Bit Set7 : simulink/Logic and Bit Operations/Bit Set  iBit=6
  Bit Set8 : simulink/Logic and Bit Operations/Bit Set  iBit=7
  Constant1 : Constant  Value=AFS_pBstLdAdjThresLo_C
  Constant2 : Constant  Value=AFS_pBstLdAdjThresHi_C
  Constant6 : Constant  Value=AFS_vVehLdAdjThresLo_C
  Constant7 : Constant  Value=AFS_vVehLdAdjThresHi_C
  Delay : Delay  DelayLength=1  InitialCondition=0
  Interval Test Dynamic1 : simulink/Logic and Bit Operations/Interval Test Dynamic  IntervalClosedRight=off  IntervalClosedLeft=off  OutDataTypeStr=boolean
  Interval Test Dynamic2 : simulink/Logic and Bit Operations/Interval Test Dynamic  IntervalClosedRight=off  IntervalClosedLeft=off  OutDataTypeStr=boolean
  Interval Test Dynamic3 : simulink/Logic and Bit Operations/Interval Test Dynamic  IntervalClosedRight=off  IntervalClosedLeft=off  OutDataTypeStr=boolean
  Logical Operator1 : Logic  Inputs=8  AllPortsSameDT=off  OutDataTypeStr=boolean
  Logical Operator3 : Logic  Operator=NOT  Inputs=5  AllPortsSameDT=off  OutDataTypeStr=boolean
  Switch{1,3..9} (8 alike) : Switch  Criteria=u2 ~= 0  OutDataTypeStr=Inherit: Inherit via back propagation  SaturateOnIntegerOverflow=on  InputSameDT=on
  stLdAdjRlsUnDeb : Outport
  wires:
  Logical Operator3/1 -> Switch8/2, Logical Operator1/7
  Logical Operator1/1 -> stLdAdjRlsUnDeb/1  "AFS_stLdAdjRlsUnDeb"
  Delay/1 -> Bit Set6/1, Bit Clear6/1
  Switch9/1 -> Delay/1  "AFS_stLdAdjRlsCon_mp"
  " LdAdjGradMon"/3(stnEngGrad) -> Switch9/2, Logical Operator1/8
  Switch8/1 -> Bit Clear8/1, Bit Set8/1
  Bit Set8/1 -> Switch9/1
  Bit Clear8/1 -> Switch9/3
  Switch7/1 -> Bit Set7/1, Bit Clear7/1
  stCurrLdAdj/1 -> Logical Operator3/1
  Bit Set7/1 -> Switch8/1
  Bit Clear7/1 -> Switch8/3
  Switch5/1 -> Bit Clear5/1, Bit Set5/1
  stAdjRlsEnvCon/1 -> Switch7/2, Logical Operator1/6
  Bit Set5/1 -> Switch7/1
  Bit Clear5/1 -> Switch7/3
  Switch4/1 -> Bit Set4/1, Bit Clear4/1
  " LdAdjGradMon"/2(stGrad) -> Switch5/2, Logical Operator1/5
  Bit Set4/1 -> Switch5/1
  Bit Clear4/1 -> Switch5/3
  Switch3/1 -> Bit Clear3/1, Bit Set3/1
  " LdAdjGradMon"/1(stBstPresGrad) -> Switch4/2, Logical Operator1/4
  Bit Set3/1 -> Switch4/1
  Bit Clear3/1 -> Switch4/3
  Switch1/1 -> Bit Set2/1, Bit Clear2/1
  Interval Test Dynamic3/1 -> Switch3/2, Logical Operator1/3
  Bit Set2/1 -> Switch3/1
  Bit Clear2/1 -> Switch3/3
  AFS_qWinLdAdjThresLo_CUR/1 -> Interval Test Dynamic3/3  "AFS_qWinLdAdjThresLo_mp"
  AFS_qWinLdAdjThresHi_CUR/1 -> Interval Test Dynamic3/1  "AFS_qWinLdAdjThresHi_mp"
  Epm_nEng/1 -> AFS_qWinLdAdjThresLo_CUR/1, " LdAdjGradMon"/2(Epm_nEng), AFS_qWinLdAdjThresHi_CUR/1
  InjCtl_qCurr/1 -> Interval Test Dynamic3/2, " LdAdjGradMon"/1(InjCtl_qCurr)
  Switch6/1 -> Bit Clear1/1, Bit Set1/1
  Interval Test Dynamic1/1 -> Switch1/2, Logical Operator1/2
  Bit Set1/1 -> Switch1/1
  Bit Clear1/1 -> Switch1/3
  ASMod_pIndVol/1 -> " LdAdjGradMon"/3(ASMod_pIndVol), Interval Test Dynamic1/2
  Constant1/1 -> Interval Test Dynamic1/3
  Constant2/1 -> Interval Test Dynamic1/1
  Interval Test Dynamic2/1 -> Logical Operator1/1, Switch6/2
  Bit Set6/1 -> Switch6/1
  Bit Clear6/1 -> Switch6/3
  VehV_v/1 -> Interval Test Dynamic2/2
  Constant6/1 -> Interval Test Dynamic2/3
  Constant7/1 -> Interval Test Dynamic2/1

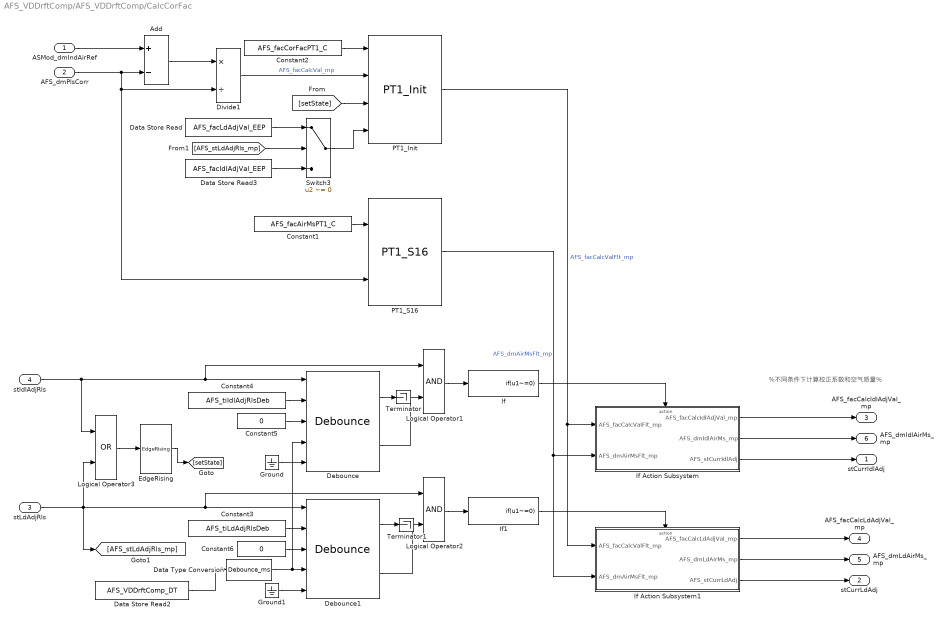
== system AFS_VDDrftComp/AFS_VDDrftComp/CalcCorFac ==
  note: %不同条件下计算校正系数和空气质量%
  ASMod_dmIndAirRef : Inport
  AFS_dmPlsCorr : Inport  Port=2
  stLdAdjRls : Inport  Port=3
  stIdlAdjRls : Inport  Port=4
  Add : Sum  Inputs=+-  OutDataTypeStr=Inherit: Inherit via back propagation  SaturateOnIntegerOverflow=on  InputSameDT=on
  Constant1 : Constant  Value=AFS_facAirMsPT1_C
  Constant2 : Constant  Value=AFS_facCorFacPT1_C
  Constant3 : Constant  Value=AFS_tiLdAdjRlsDeb
  Constant4 : Constant  Value=AFS_tiIdlAdjRlsDeb
  Constant5 : Constant  Value=0  OutDataTypeStr=Debounce_ms
  Constant6 : Constant  Value=0  OutDataTypeStr=Debounce_ms
  Data Store Read : DataStoreRead  DataStoreName=AFS_facLdAdjVal_EEP
  Data Store Read2 : DataStoreRead  DataStoreName=AFS_VDDrftComp_DT
  Data Store Read3 : DataStoreRead  DataStoreName=AFS_facIdlAdjVal_EEP
  Data Type Conversion : DataTypeConversion  OutDataTypeStr=Debounce_ms
  Debounce : CXLib/Debounce
  Debounce1 : CXLib/Debounce
  Divide1 : Product  Inputs=*/  OutDataTypeStr=Inherit: Inherit via back propagation  SaturateOnIntegerOverflow=on  InputSameDT=on
  EdgeRising : CXLib/EdgeRising
  Ground : Ground
  Ground1 : Ground
  If : If  IfExpression=u1~=0  ShowElse=off
  If Action Subsystem : Subsystem  TreatAsAtomicUnit=on
  If Action Subsystem1 : Subsystem  TreatAsAtomicUnit=on
  If1 : If  IfExpression=u1~=0  ShowElse=off
  Logical Operator1 : Logic  OutDataTypeStr=boolean
  Logical Operator2 : Logic  OutDataTypeStr=boolean
  Logical Operator3 : Logic  Operator=OR  OutDataTypeStr=boolean
  PT1_Init : CXLib/PT1_Init
  PT1_S16 : CXLib/PT1_S16
  Switch3 : Switch  Criteria=u2 ~= 0  OutDataTypeStr=Inherit: Inherit via back propagation  SaturateOnIntegerOverflow=on  InputSameDT=on
  Terminator : Terminator
  Terminator1 : Terminator
  stCurrIdlAdj : Outport
  stCurrLdAdj : Outport  Port=2
  AFS_facCalcIdlAdjVal_mp : Outport  Port=3
  AFS_facCalcLdAdjVal_mp : Outport  Port=4
  AFS_dmLdAirMs_mp : Outport  Port=5
  AFS_dmIdlAirMs_mp : Outport  Port=6
  wires:
  Debounce1/2 -> Logical Operator2/2
  Debounce1/1 -> Terminator1/1
  Debounce/1 -> Terminator/1
  If Action Subsystem1/3(AFS_stCurrLdAdj) -> stCurrLdAdj/1
  If Action Subsystem1/2(AFS_dmLdAirMs_mp) -> AFS_dmLdAirMs_mp/1
  If Action Subsystem1/1(AFS_facCalcLdAdjVal_mp) -> AFS_facCalcLdAdjVal_mp/1
  If Action Subsystem/2(AFS_dmIdlAirMs_mp) -> AFS_dmIdlAirMs_mp/1
  If Action Subsystem/1(AFS_facCalcIdlAdjVal_mp) -> AFS_facCalcIdlAdjVal_mp/1
  If Action Subsystem/3(AFS_stCurrIdlAdj) -> stCurrIdlAdj/1
  PT1_S16/1 -> If Action Subsystem1/2(AFS_dmAirMsFlt_mp), If Action Subsystem/2(AFS_dmAirMsFlt_mp)  "AFS_dmAirMsFlt_mp"
  PT1_Init/1 -> If Action Subsystem/1(AFS_facCalcValFlt_mp), If Action Subsystem1/1(AFS_facCalcValFlt_mp)  "AFS_facCalcValFlt_mp"
  If1/1 -> If Action Subsystem1/Action
  [AFS_stLdAdjRls_mp] -> Switch3/2
  [setState] -> PT1_Init/3
  EdgeRising/1 -> [setState]
  Logical Operator3/1 -> EdgeRising/1
  Switch3/1 -> PT1_Init/4
  Data Store Read3/1 -> Switch3/3
  Data Store Read/1 -> Switch3/1
  If/1 -> If Action Subsystem/Action
  Logical Operator2/1 -> If1/1
  Constant6/1 -> Debounce1/3
  Constant3/1 -> Debounce1/2
  Data Store Read2/1 -> Data Type Conversion/1
  Ground1/1 -> Debounce1/5
  stLdAdjRls/1 -> Logical Operator3/2, Logical Operator2/1, Debounce1/1, [AFS_stLdAdjRls_mp]
  Logical Operator1/1 -> If/1
  Debounce/2 -> Logical Operator1/2
  Constant5/1 -> Debounce/3
  Constant4/1 -> Debounce/2
  Data Type Conversion/1 -> Debounce/4, Debounce1/4
  Ground/1 -> Debounce/5
  stIdlAdjRls/1 -> Logical Operator3/1, Debounce/1, Logical Operator1/1
  Constant1/1 -> PT1_S16/1
  Constant2/1 -> PT1_Init/1
  Divide1/1 -> PT1_Init/2  "AFS_facCalcVal_mp"
  Add/1 -> Divide1/1
  AFS_dmPlsCorr/1 -> Add/2, Divide1/2, PT1_S16/2
  ASMod_dmIndAirRef/1 -> Add/1

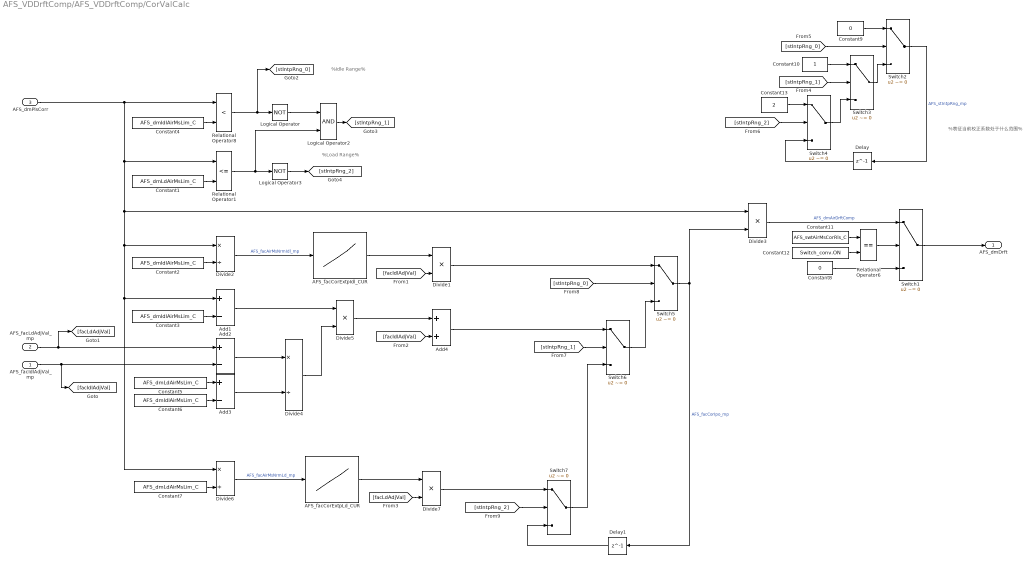
== system AFS_VDDrftComp/AFS_VDDrftComp/CorValCalc ==
  note: %Idle Range%
  note: %Load Range%
  note: %表征当前校正系数处于什么范围%
  AFS_facIdlAdjVal_mp : Inport
  AFS_facLdAdjVal_mp : Inport  Port=2
  AFS_dmPlsCorr : Inport  Port=3
  AFS_facCorExtpIdl_CUR : Lookup_n-D  NumberOfTableDimensions=1  BreakpointsForDimension1=AFS_facCorExtpIdl_CURX  IndexSearchMethod=Linear search  BeginIndexSearchUsingPreviousIndexResult=on  UseOneInputPortForAllInputData=on  Table=AFS_facCorExtpIdl_CUR  ExtrapMethod=Clip  UseLastTableValue=on  InternalRulePriority=Speed  OutDataTypeStr=Inherit: Inherit via back propagation  SaturateOnIntegerOverflow=on
  AFS_facCorExtpLd_CUR : Lookup_n-D  NumberOfTableDimensions=1  BreakpointsForDimension1=AFS_facCorExtpLd_CURX  IndexSearchMethod=Linear search  BeginIndexSearchUsingPreviousIndexResult=on  UseOneInputPortForAllInputData=on  Table=AFS_facCorExtpLd_CUR  ExtrapMethod=Clip  UseLastTableValue=on  InternalRulePriority=Speed  OutDataTypeStr=Inherit: Inherit via back propagation  SaturateOnIntegerOverflow=on
  Add1 : Sum  Inputs=+-  OutDataTypeStr=Inherit: Inherit via back propagation  SaturateOnIntegerOverflow=on  InputSameDT=on
  Add2 : Sum  Inputs=+-  OutDataTypeStr=Inherit: Inherit via back propagation  SaturateOnIntegerOverflow=on  InputSameDT=on
  Add3 : Sum  Inputs=+-  SaturateOnIntegerOverflow=on  InputSameDT=on  OutDataTypeStr=Inherit: Same as first input
  Add4 : Sum  OutDataTypeStr=Inherit: Inherit via back propagation  SaturateOnIntegerOverflow=on  InputSameDT=on
  Constant1 : Constant  Value=AFS_dmLdAirMsLim_C
  Constant10 : Constant  OutDataTypeStr=Inherit: Inherit via back propagation
  Constant11 : Constant  Value=AFS_swtAirMsCorRls_C
  Constant12 : Constant  Value=Switch_conv.ON
  Constant13 : Constant  Value=2  OutDataTypeStr=Inherit: Inherit via back propagation
  Constant{2..4,6} (4 alike) : Constant  Value=AFS_dmIdlAirMsLim_C
  Constant5 : Constant  Value=AFS_dmLdAirMsLim_C
  Constant7 : Constant  Value=AFS_dmLdAirMsLim_C
  Constant8 : Constant  Value=0  OutDataTypeStr=Inherit: Inherit via back propagation
  Constant9 : Constant  Value=0  OutDataTypeStr=Inherit: Inherit via back propagation
  Delay : Delay  DelayLength=1  InitialCondition=0
  Delay1 : Delay  DelayLength=1  InitialCondition=0
  Divide{1,3,5,7} (4 alike) : Product  Inputs=**  OutDataTypeStr=Inherit: Inherit via back propagation  SaturateOnIntegerOverflow=on
  Divide2 : Product  Inputs=*/  OutDataTypeStr=Inherit: Inherit via back propagation  SaturateOnIntegerOverflow=on
  Divide4 : Product  Inputs=*/  SaturateOnIntegerOverflow=on
  Divide6 : Product  Inputs=*/  OutDataTypeStr=Inherit: Inherit via back propagation  SaturateOnIntegerOverflow=on
  Logical Operator : Logic  Operator=NOT  AllPortsSameDT=off  OutDataTypeStr=boolean
  Logical Operator2 : Logic  OutDataTypeStr=boolean
  Logical Operator3 : Logic  Operator=NOT  AllPortsSameDT=off  OutDataTypeStr=boolean
  Relational Operator1 : RelationalOperator  Operator=<=  OutDataTypeStr=boolean  RndMeth=Simplest  InputSameDT=on
  Relational Operator6 : RelationalOperator  Operator===  OutDataTypeStr=boolean  RndMeth=Simplest
  Relational Operator8 : RelationalOperator  Operator=<  OutDataTypeStr=boolean  RndMeth=Simplest  InputSameDT=on
  Switch{1..7} (7 alike) : Switch  Criteria=u2 ~= 0  OutDataTypeStr=Inherit: Inherit via back propagation  SaturateOnIntegerOverflow=on  InputSameDT=on
  AFS_dmDrft : Outport
  wires:
  Delay1/1 -> Switch7/3
  Divide7/1 -> Switch7/1
  [stIntpRng_2] -> Switch7/2
  Switch7/1 -> Switch6/3
  Add4/1 -> Switch6/1
  [stIntpRng_1] -> Switch6/2
  Switch6/1 -> Switch5/3
  Divide1/1 -> Switch5/1
  [stIntpRng_0] -> Switch5/2
  Switch5/1 -> Divide3/2, Delay1/1  "AFS_facCorIpo_mp"
  [facIdlAdjVal] -> Divide1/2
  [facLdAdjVal] -> Divide7/2
  Delay/1 -> Switch4/3
  Constant13/1 -> Switch4/1
  [stIntpRng_2] -> Switch4/2
  Switch4/1 -> Switch3/3
  Constant10/1 -> Switch3/1
  [stIntpRng_1] -> Switch3/2
  Switch3/1 -> Switch2/3
  Constant9/1 -> Switch2/1
  [stIntpRng_0] -> Switch2/2
  Switch2/1 -> Delay/1  "AFS_stIntpRng_mp"
  Logical Operator3/1 -> [stIntpRng_2]
  AFS_facLdAdjVal_mp/1 -> [facLdAdjVal], Add2/1
  Switch1/1 -> AFS_dmDrft/1
  Constant8/1 -> Switch1/3
  Relational Operator6/1 -> Switch1/2
  Constant11/1 -> Relational Operator6/1
  Constant12/1 -> Relational Operator6/2
  AFS_facCorExtpLd_CUR/1 -> Divide7/1
  Divide6/1 -> AFS_facCorExtpLd_CUR/1  "AFS_facAirMsNrmLd_mp"
  Constant7/1 -> Divide6/2
  [facIdlAdjVal] -> Add4/2
  Divide5/1 -> Add4/1
  Divide4/1 -> Divide5/2
  Add1/1 -> Divide5/1
  Add3/1 -> Divide4/2
  Constant6/1 -> Add3/2
  Constant5/1 -> Add3/1
  Add2/1 -> Divide4/1
  AFS_facIdlAdjVal_mp/1 -> [facIdlAdjVal], Add2/2
  Constant3/1 -> Add1/2
  Divide3/1 -> Switch1/1  "AFS_dmAirDrftComp"
  AFS_dmPlsCorr/1 -> Relational Operator8/1, Relational Operator1/1, Divide2/1, Add1/1, Divide6/1, Divide3/1
  Logical Operator2/1 -> [stIntpRng_1]
  Relational Operator1/1 -> Logical Operator2/2, Logical Operator3/1
  Logical Operator/1 -> Logical Operator2/1
  AFS_facCorExtpIdl_CUR/1 -> Divide1/1
  Divide2/1 -> AFS_facCorExtpIdl_CUR/1  "AFS_facAirMsNrmIdl_mp"
  Constant2/1 -> Divide2/2
  Relational Operator8/1 -> Logical Operator/1, [stIntpRng_0]
  Constant1/1 -> Relational Operator1/2
  Constant4/1 -> Relational Operator8/2

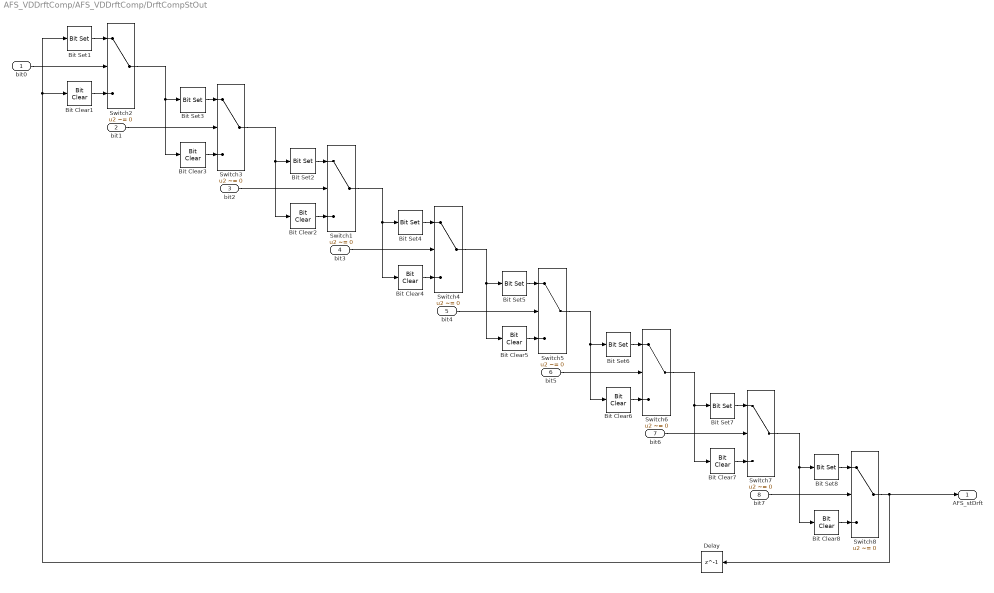
== system AFS_VDDrftComp/AFS_VDDrftComp/DrftCompStOut ==
  bit0 : Inport
  bit1 : Inport  Port=2
  bit2 : Inport  Port=3
  bit3 : Inport  Port=4
  bit4 : Inport  Port=5
  bit5 : Inport  Port=6
  bit6 : Inport  Port=7
  bit7 : Inport  Port=8
  Bit Clear1 : simulink/Logic and Bit Operations/Bit Clear  iBit=0
  Bit Clear2 : simulink/Logic and Bit Operations/Bit Clear  iBit=2
  Bit Clear3 : simulink/Logic and Bit Operations/Bit Clear  iBit=1
  Bit Clear4 : simulink/Logic and Bit Operations/Bit Clear  iBit=3
  Bit Clear5 : simulink/Logic and Bit Operations/Bit Clear  iBit=4
  Bit Clear6 : simulink/Logic and Bit Operations/Bit Clear  iBit=5
  Bit Clear7 : simulink/Logic and Bit Operations/Bit Clear  iBit=6
  Bit Clear8 : simulink/Logic and Bit Operations/Bit Clear  iBit=7
  Bit Set1 : simulink/Logic and Bit Operations/Bit Set  iBit=0
  Bit Set2 : simulink/Logic and Bit Operations/Bit Set  iBit=2
  Bit Set3 : simulink/Logic and Bit Operations/Bit Set  iBit=1
  Bit Set4 : simulink/Logic and Bit Operations/Bit Set  iBit=3
  Bit Set5 : simulink/Logic and Bit Operations/Bit Set  iBit=4
  Bit Set6 : simulink/Logic and Bit Operations/Bit Set  iBit=5
  Bit Set7 : simulink/Logic and Bit Operations/Bit Set  iBit=6
  Bit Set8 : simulink/Logic and Bit Operations/Bit Set  iBit=7
  Delay : Delay  DelayLength=1  InitialCondition=0
  Switch{1..8} (8 alike) : Switch  Criteria=u2 ~= 0  OutDataTypeStr=Inherit: Inherit via back propagation  SaturateOnIntegerOverflow=on  InputSameDT=on
  AFS_stDrft : Outport
  wires:
  Delay/1 -> Bit Clear1/1, Bit Set1/1
  Switch8/1 -> AFS_stDrft/1, Delay/1
  bit7/1 -> Switch8/2
  Switch7/1 -> Bit Clear8/1, Bit Set8/1
  Bit Clear8/1 -> Switch8/3
  Bit Set8/1 -> Switch8/1
  bit6/1 -> Switch7/2
  Switch6/1 -> Bit Set7/1, Bit Clear7/1
  Bit Clear7/1 -> Switch7/3
  Bit Set7/1 -> Switch7/1
  bit5/1 -> Switch6/2
  Switch5/1 -> Bit Clear6/1, Bit Set6/1
  Bit Clear6/1 -> Switch6/3
  Bit Set6/1 -> Switch6/1
  bit4/1 -> Switch5/2
  Switch4/1 -> Bit Set5/1, Bit Clear5/1
  Bit Clear5/1 -> Switch5/3
  Bit Set5/1 -> Switch5/1
  bit3/1 -> Switch4/2
  Switch1/1 -> Bit Clear4/1, Bit Set4/1
  Bit Clear4/1 -> Switch4/3
  Bit Set4/1 -> Switch4/1
  bit2/1 -> Switch1/2
  Switch3/1 -> Bit Set2/1, Bit Clear2/1
  Bit Clear2/1 -> Switch1/3
  Bit Set2/1 -> Switch1/1
  bit1/1 -> Switch3/2
  Bit Clear1/1 -> Switch2/3
  Switch2/1 -> Bit Clear3/1, Bit Set3/1
  Bit Clear3/1 -> Switch3/3
  Bit Set3/1 -> Switch3/1
  Bit Set1/1 -> Switch2/1
  bit0/1 -> Switch2/2

== system AFS_VDDrftComp/AFS_VDDrftComp/EGRClsDem ==
  note: %Request for closing the exhaust gas recirculation valve %
  AirCtl_stMon : Inport
  stIdlAdjRlsUnDeb : Inport  Port=2
  stLdAdjRlsUnDeb : Inport  Port=3
  Constant1 : Constant  Value=true  OutDataTypeStr=boolean
  Constant2 : Constant  Value=AIRCTL_DRFTCOMP  OutDataTypeStr=Inherit: Inherit via back propagation
  Constant5 : Constant  Value=AFS_tiAdjRlsDel_C
  Data Store Read : DataStoreRead  DataStoreName=AFS_VDDrftComp_DT
  Data Type Conversion : DataTypeConversion
  Delay : Delay  DelayLength=1  InitialCondition=0
  Logical Operator{,3..5} (4 alike) : Logic  OutDataTypeStr=boolean
  Logical Operator1 : Logic  Operator=OR  OutDataTypeStr=boolean
  Logical Operator2 : Logic  Operator=NOT  AllPortsSameDT=off  OutDataTypeStr=boolean
  Relational Operator : RelationalOperator  Operator===  OutDataTypeStr=boolean  ZeroCross=off  RndMeth=Simplest  InputSameDT=on
  Switch6 : Switch  Criteria=u2 ~= 0  OutDataTypeStr=Inherit: Inherit via back propagation  SaturateOnIntegerOverflow=on  InputSameDT=on
  TurnOnDelay : CXLib/TurnOnDelay
  stLdAdjRls : Outport
  stIdlAdjRls : Outport  Port=2
  stEGRClsDem : Outport  Port=3
  wires:
  Logical Operator5/1 -> stIdlAdjRls/1  "AFS_stIdlAdjRls"
  Logical Operator4/1 -> stLdAdjRls/1  "AFS_stLdAdjRls"
  Delay/1 -> Switch6/2
  Logical Operator3/1 -> Delay/1
  Logical Operator2/1 -> Logical Operator3/2
  Logical Operator/1 -> TurnOnDelay/1, Logical Operator3/1
  Relational Operator/1 -> Logical Operator/2
  Switch6/1 -> Logical Operator/1, stEGRClsDem/1
  Constant1/1 -> Switch6/1
  Logical Operator1/1 -> Switch6/3
  stLdAdjRlsUnDeb/1 -> Logical Operator1/2, Logical Operator4/2
  stIdlAdjRlsUnDeb/1 -> Logical Operator1/1, Logical Operator5/2
  TurnOnDelay/1 -> Logical Operator2/1, Logical Operator4/1, Logical Operator5/1  "AFS_stAdjRlsDel_mp"
  Constant5/1 -> TurnOnDelay/2
  AirCtl_stMon/1 -> Relational Operator/1
  Constant2/1 -> Relational Operator/2
  Data Store Read/1 -> Data Type Conversion/1
  Data Type Conversion/1 -> TurnOnDelay/3
